simulink library "util_event_lib"  (R2014b)
settings: Solver=ode45  StartTime=0.0  StopTime=10.0  RelTol=1e-3
libraries: util_info_lib x1
settings Model: Creator=mstewart  LastModifiedBy=mstewart

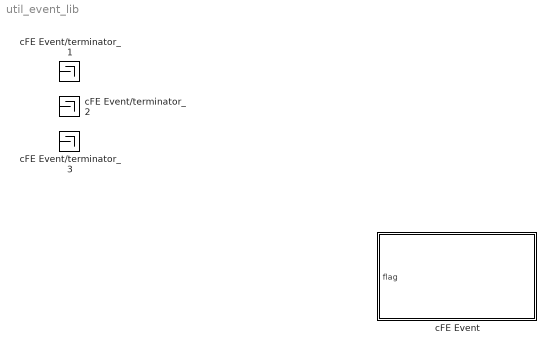
== system util_event_lib ==
  cFE Event : Subsystem  TreatAsAtomicUnit=on  mask{event_message='Sample Message \n', event_id=0, event_severity=DEBUG, event_filtered=off, event_mask=1, event_use_enums=off, event_enum_types={}}
      mask prompts: event_message "Event Message (include ')"; event_id "Event ID"; event_severity "Severity"; event_filtered "Filter Event"; event_mask "Event FIltering Mask"; event_use_enums "Use Enumerated Inputs"; event_enum_types "Enumeration Types"
      mask help:
      | Sends a cFE event when the 'flag' input is high.
      |
      | The Event Message field is a standard printf-formatted string. This block will automatically adjust its number of inputs based on the format of the string. String formatting tokens (%s) are only supported for enumerated inputs.
      |
      | To use enumerated inputs, check the "Use Enumerated Inputs" block. The Enumeration Types field must then be set to a 1xN cell array of strings, where N is the number of data inputs to the block (not including the flag). Each string in the cell array should be the name of enumeration used for the corresponding input. Non-enumerated inputs should be entered as an empty string.
      mask init:
      | util_event_callback(gcb, event_message, event_id, event_severity, event_filtered, event_mask, event_use_enums, event_enum_types);
      settings: RTWSystemCode=Inline
      mask TypeOptions event_severity: DEBUG | INFORMATION | ERROR | CRITICAL
      mask Callback event_filtered: mask_checkbox_set_param_enabled(gcb, 'event_filtered', 'event_mask')
      mask Callback event_use_enums: mask_checkbox_set_param_enabled(gcb, 'event_use_enums', 'event_enum_types')
      mask Display:
      | disp('Send Event');
      | color('blue');
      | text(0.05,0.02,'MoonEx', ...
      |     'HorizontalAlignment', 'Left', ...
      |     'VerticalAlignment', 'Bottom');
  cFE Event/terminator_1 : Terminator
  cFE Event/terminator_2 : Terminator
  cFE Event/terminator_3 : Terminator

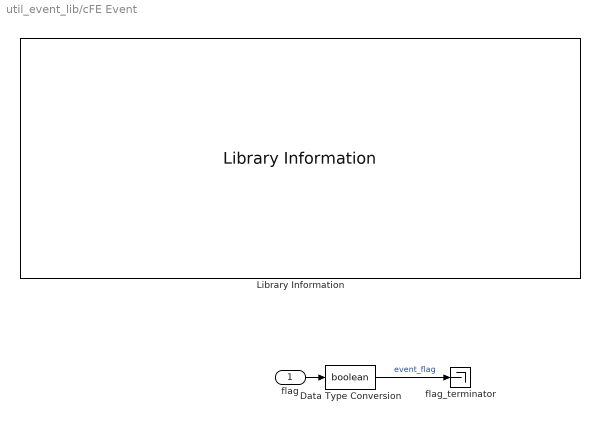
== system util_event_lib/cFE Event ==
  flag : Inport
  Data Type Conversion : DataTypeConversion  OutDataTypeStr=boolean
  Library Information : util_info_lib/Library Information  owner='NONE'
  flag_terminator : Terminator
  wires:
  flag/1 -> Data Type Conversion/1
  Data Type Conversion/1 -> flag_terminator/1  "event_flag"
